simulink model "RLC"  (R2015a)
settings: Solver=ode4  StartTime=0.0  StopTime=5  FixedStep=0.0001  RelTol=1e-3
settings Model: Creator=Anirudh  LastModifiedBy=Aranya Dan

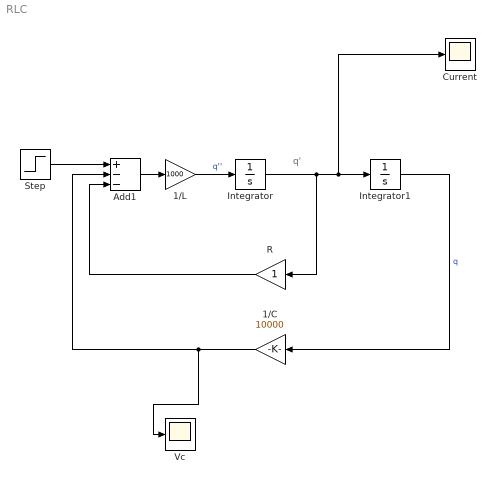
== system RLC ==
  note: q'
  1/C : Gain  Gain=10000
  1/L : Gain  Gain=1000
  Add1 : Sum  Inputs=+--
  Current : Scope
      settings: SaveName=ScopeData2
  Integrator : Integrator
  Integrator1 : Integrator
  R : Gain
  Step : Step  Time=0  After=10  SampleTime=0
  Vc : Scope
  wires:
  Integrator1/1 -> 1/C/1  "q"
  Integrator/1 -> R/1, Current/1, Integrator1/1
  Add1/1 -> 1/L/1
  R/1 -> Add1/3
  1/C/1 -> Vc/1, Add1/2
  Step/1 -> Add1/1
  1/L/1 -> Integrator/1  "q''"
